simulink model "lab5_sim"  (R2021b)
settings: Solver=VariableStepAuto  StartTime=0.0  StopTime=10.0  RelTol=1e-3
values from neighbouring files (symbols this model uses):
  C = eye(4)    [lab5.m]    (also in lab5_2.m)
  D = [0;0;0;0]    [lab5.m]    (also in lab5_2.m)
  multi_step = [1;0;0;0]    [lab5_2.m]
undefined symbols (not defined in the file or in its folder): A_a, A_b, A_c, B_a, B_b, B_c
libraries: truetime x1
settings Model: Creator=varunsampat  LastModifiedBy=varunsampat

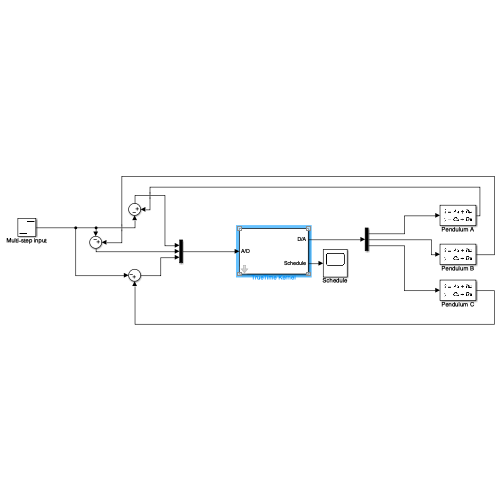
[thumbnail: Simulink's stored preview of the top-level diagram]
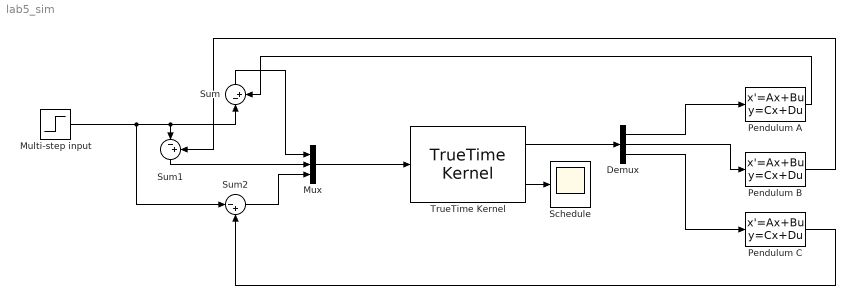
== system lab5_sim ==
  Demux : Demux  Outputs=3
  Multi-step input : Step  Before=zeros(4,1)  After=multi_step  SampleTime=0
  Mux : Mux  Inputs=3
  Pendulum A : StateSpace  A=A_a  B=B_a  C=C  D=D  InitialCondition=0
  Pendulum B : StateSpace  A=A_b  B=B_b  C=C  D=D  InitialCondition=0
  Pendulum C : StateSpace  A=A_c  B=B_c  C=C  D=D  InitialCondition=0
  Schedule : Scope
  Sum : Sum  Inputs=|-+
  Sum1 : Sum  Inputs=|-+
  Sum2 : Sum  Inputs=|-+
  TrueTime Kernel : truetime/TrueTime Kernel  sfun=node_init  args=[]  ninputsoutputs=[12 3]  ntriggers=0  trigtype=falling  nwnodenbr=[]  clockoffsetdrift=[0 0]  schedoutput=on  battery=off  poweroutput=off
  wires:
  Pendulum A/1 -> Sum/2
  Pendulum B/1 -> Sum1/2
  Pendulum C/1 -> Sum2/2
  TrueTime Kernel/2 -> Schedule/1
  Multi-step input/1 -> Sum2/1, Sum/1, Sum1/1
  TrueTime Kernel/1 -> Demux/1
  Mux/1 -> TrueTime Kernel/1
  Sum/1 -> Mux/1
  Sum1/1 -> Mux/2
  Sum2/1 -> Mux/3
  Demux/1 -> Pendulum A/1
  Demux/3 -> Pendulum C/1
  Demux/2 -> Pendulum B/1
